simulink model "HW3"  (R2018a)
settings: Solver=VariableStepAuto  StartTime=0.0  StopTime=2400  RelTol=1e-3
settings Model: Creator=rahul  LastModifiedBy=rahul

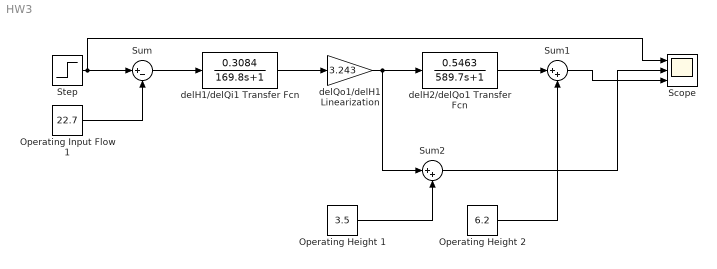
== system HW3 ==
  Operating Height 1 : Constant  Value=3.5
  Operating Height 2 : Constant  Value=6.2
  Operating Input Flow 1 : Constant  Value=22.7
  Scope : Scope  NumInputPorts=3
  "Step " : Step  Before=22.7  After=24.3  SampleTime=0
  Sum : Sum  Inputs=|+-
  Sum1 : Sum  Inputs=|++
  Sum2 : Sum  Inputs=|++
  delH1/delQi1 Transfer Fcn : TransferFcn  Numerator=0.3084  Denominator=[169.8 1]
  delH2/delQo1 Transfer Fcn : TransferFcn  Numerator=[0.5463]  Denominator=[589.7 1]
  "delQo1/delH1 Linearization " : Gain  Gain=3.243
  wires:
  delH1/delQi1 Transfer Fcn/1 -> "delQo1/delH1 Linearization "/1
  Sum/1 -> delH1/delQi1 Transfer Fcn/1
  delH2/delQo1 Transfer Fcn/1 -> Sum1/1
  "delQo1/delH1 Linearization "/1 -> Sum2/1, delH2/delQo1 Transfer Fcn/1
  "Step "/1 -> Scope/1, Sum/1
  Operating Input Flow 1/1 -> Sum/2
  Operating Height 1/1 -> Sum2/2
  Operating Height 2/1 -> Sum1/2
  Sum2/1 -> Scope/2
  Sum1/1 -> Scope/3
